simulink model "ADCS_GNC_Real_Simulation"  (R2025a)
settings: Solver=ode4  StartTime=0.0  StopTime=600  FixedStep=dt_sim  RelTol=1e-3
values from neighbouring files (symbols this model uses):
  Area_drag = 1.5    [ADCS_Real_Baseline.m]    (also in ADCS_Real_Baseline_Aerospace_Toolbox.m)
  Cd = 2.2    [ADCS_Real_Baseline.m]    (also in ADCS_Real_Baseline_Aerospace_Toolbox.m)
  cp_cg_offset_drag = [0.05; 0.02; -0.03]    [ADCS_Real_Baseline.m]    (also in ADCS_Real_Baseline_Aerospace_Toolbox.m)
  g0 = 9.80665    [ADCS_Real_Baseline.m]    (also in ADCS_Real_Baseline_Aerospace_Toolbox.m)
  gyro_bias_true = [1e-4; -2e-4; 1.5e-4]    [ADCS_Real_Baseline.m]    (also in ADCS_Real_Baseline_Aerospace_Toolbox.m)
  gyro_noise_sigma = 1e-5    (= 1e-05)    [ADCS_Real_Baseline.m]    (also in ADCS_Real_Baseline_Aerospace_Toolbox.m)
  I_inv = inv(I_tensor)    [ADCS_Real_Baseline.m]    (also in ADCS_Real_Baseline_Aerospace_Toolbox.m)
  I_tensor = diag([I_xx, I_yy, I_zz])    [ADCS_Real_Baseline.m]    (also in ADCS_Real_Baseline_Aerospace_Toolbox.m)
  Kd = diag(diag(2 * zeta * I_tensor * omega_n))    [ADCS_Real_Baseline.m]    (also in ADCS_Real_Baseline_Aerospace_Toolbox.m)
  Kp = diag(diag(I_tensor * omega_n^2))    [ADCS_Real_Baseline.m]    (also in ADCS_Real_Baseline_Aerospace_Toolbox.m)
  mtq_max_dipole = 15.0    (= 15)    [ADCS_Real_Baseline.m]    (also in ADCS_Real_Baseline_Aerospace_Toolbox.m)
  mtq_power_W_per_Am2 = 0.5    [ADCS_Real_Baseline.m]    (also in ADCS_Real_Baseline_Aerospace_Toolbox.m)
  mu_E = 398600.4418    [ADCS_Real_Baseline.m]    (also in ADCS_Real_Baseline_Aerospace_Toolbox.m)
  omega_init = C_BL_init * omega_orb_LVLH    [ADCS_Real_Baseline.m]    (also in ADCS_Real_Baseline_Aerospace_Toolbox.m)
  omega_orb_mag = sqrt(mu_E / r_orbit^3)    [ADCS_Real_Baseline.m]    (also in ADCS_Real_Baseline_Aerospace_Toolbox.m)
  q_init = q_init / norm(q_init)    [ADCS_Real_Baseline.m]    (also in ADCS_Real_Baseline_Aerospace_Toolbox.m)
  q_LVLH_ECI_init = q_LVLH_ECI_init / norm(q_LVLH_ECI_init)    [ADCS_Real_Baseline.m]    (also in ADCS_Real_Baseline_Aerospace_Toolbox.m)
  r_orbit = R_E + h_orbit    (= 7171)    [ADCS_Real_Baseline.m]    (also in ADCS_Real_Baseline_Aerospace_Toolbox.m)
  rho_atm = 1e-13    [ADCS_Real_Baseline.m]    (also in ADCS_Real_Baseline_Aerospace_Toolbox.m)
  rw_max_torque = 0.05    [ADCS_Real_Baseline.m]    (also in ADCS_Real_Baseline_Aerospace_Toolbox.m)
  rw_power_W_per_Nm = 50.0    (= 50)    [ADCS_Real_Baseline.m]    (also in ADCS_Real_Baseline_Aerospace_Toolbox.m)
  st_noise_sigma = 5e-4    (= 0.0005)    [ADCS_Real_Baseline.m]    (also in ADCS_Real_Baseline_Aerospace_Toolbox.m)
  thruster_arm = 0.5    [ADCS_Real_Baseline.m]    (also in ADCS_Real_Baseline_Aerospace_Toolbox.m)
  thruster_Isp = 65.0    (= 65)    [ADCS_Real_Baseline.m]    (also in ADCS_Real_Baseline_Aerospace_Toolbox.m)
  thruster_max_torque = thruster_force * thruster_arm    (= 0.5)    [ADCS_Real_Baseline.m]    (also in ADCS_Real_Baseline_Aerospace_Toolbox.m)
  V_orb = sqrt(mu_E*1e9 / (r_orbit*1e3))    [ADCS_Real_Baseline.m]    (also in ADCS_Real_Baseline_Aerospace_Toolbox.m)
(part 1 of 2)
settings Model: Creator=Simone  LastModifiedBy=Simone

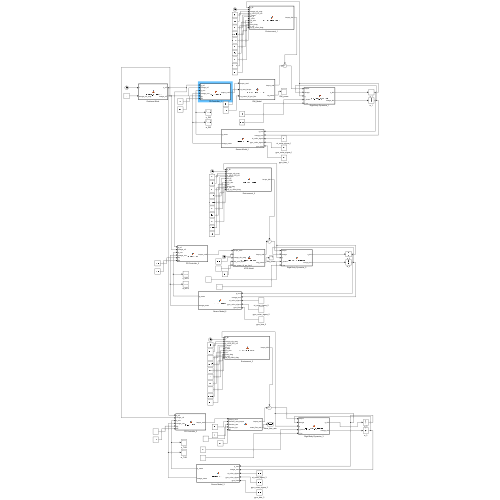
[thumbnail: Simulink's stored preview of the top-level diagram]
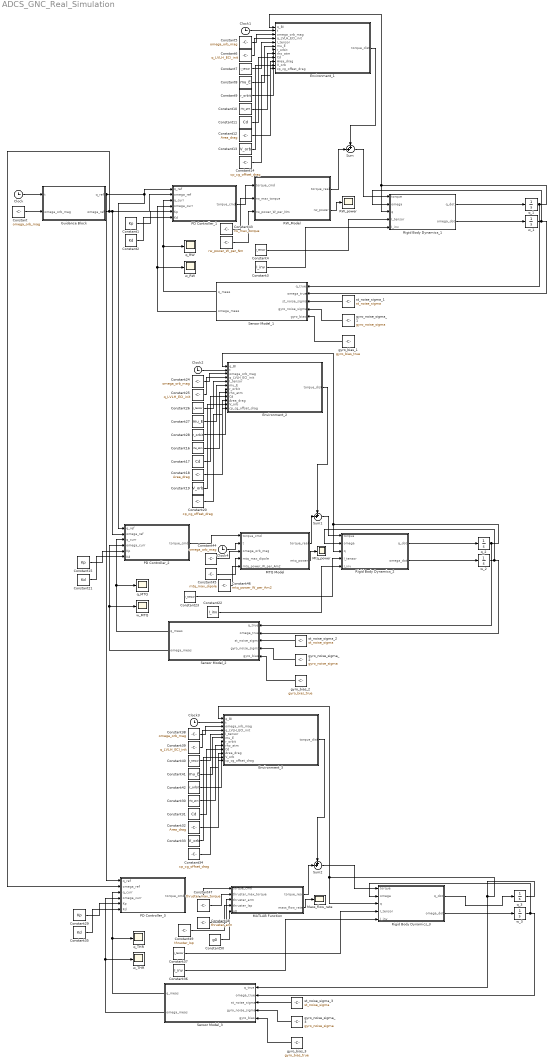
== system ADCS_GNC_Real_Simulation ==
  "                   " : Constant  Value=rw_power_W_per_Nm
  Clock{,1..4} (5 alike) : Clock
  Constant{,5,24,38,44} (5 alike) : Constant  Value=omega_orb_mag
  Constant1 : Constant  Value=Kp
  Constant10 : Constant  Value=rho_atm
  Constant11 : Constant  Value=Cd
  Constant12 : Constant  Value=Area_drag
  Constant13 : Constant  Value=V_orb
  Constant14 : Constant  Value=cp_cg_offset_drag
  Constant15 : Constant  Value=Kp
  Constant16 : Constant  Value=rho_atm
  Constant17 : Constant  Value=Cd
  Constant18 : Constant  Value=Area_drag
  Constant19 : Constant  Value=V_orb
  Constant2 : Constant  Value=Kd
  Constant20 : Constant  Value=cp_cg_offset_drag
  Constant21 : Constant  Value=Kd
  Constant22 : Constant  Value=I_inv
  Constant{4,7,23,26,37,40} (6 alike) : Constant  Value=I_tensor
  Constant25 : Constant  Value=q_LVLH_ECI_init
  Constant27 : Constant  Value=mu_E
  Constant28 : Constant  Value=r_orbit
  Constant29 : Constant  Value=Kp
  Constant3 : Constant  Value=I_inv
  Constant30 : Constant  Value=rho_atm
  Constant31 : Constant  Value=Cd
  Constant32 : Constant  Value=Area_drag
  Constant33 : Constant  Value=V_orb
  Constant34 : Constant  Value=cp_cg_offset_drag
  Constant35 : Constant  Value=Kd
  Constant36 : Constant  Value=I_inv
  Constant39 : Constant  Value=q_LVLH_ECI_init
  Constant41 : Constant  Value=mu_E
  Constant42 : Constant  Value=r_orbit
  Constant43 : Constant  Value=rw_max_torque
  Constant45 : Constant  Value=mtq_max_dipole
  Constant46 : Constant  Value=mtq_power_W_per_Am2
  Constant47 : Constant  Value=thruster_max_torque
  Constant48 : Constant  Value=thruster_arm
  Constant49 : Constant  Value=thruster_Isp
  Constant50 : Constant  Value=g0
  Constant6 : Constant  Value=q_LVLH_ECI_init
  Constant8 : Constant  Value=mu_E
  Constant9 : Constant  Value=r_orbit
  Environment_1 : MATLAB Function  TreatAsAtomicUnit=on
  Environment_2 : MATLAB Function  TreatAsAtomicUnit=on
  Environment_3 : MATLAB Function  TreatAsAtomicUnit=on
  Guidance Block : MATLAB Function  TreatAsAtomicUnit=on
  MATLAB Function : MATLAB Function  TreatAsAtomicUnit=on
  MTQ Model : MATLAB Function  TreatAsAtomicUnit=on
  Mass_flow_rate : Scope
      settings: ActiveDisplayYMinimum=-1  ActiveDisplayYMaximum=1  DataLoggingVariableName=out_mass_THR
  Mtq_power : Scope
      settings: ActiveDisplayYMinimum=-2.7921062281111855  ActiveDisplayYMaximum=25.310234025345686  DataLoggingVariableName=out_pwr_MTQ
  PD Controller_1 : MATLAB Function  TreatAsAtomicUnit=on
  PD Controller_2 : MATLAB Function  TreatAsAtomicUnit=on
  PD Controller_3 : MATLAB Function  TreatAsAtomicUnit=on
  RW_Model : MATLAB Function  TreatAsAtomicUnit=on
  RW_power : Scope
      settings: ActiveDisplayYMinimum=-0.049707954555951867  ActiveDisplayYMaximum=0.450202323670987  DataLoggingVariableName=out_pwr_RW
  Rigid Body Dynamics_1 : MATLAB Function  TreatAsAtomicUnit=on
  Rigid Body Dynamics_2 : MATLAB Function  TreatAsAtomicUnit=on
  Rigid Body Dynamics_3 : MATLAB Function  TreatAsAtomicUnit=on
  Sensor Model_1 : MATLAB Function  TreatAsAtomicUnit=on
  Sensor Model_2 : MATLAB Function  TreatAsAtomicUnit=on
  Sensor Model_3 : MATLAB Function  TreatAsAtomicUnit=on
  Sum : Sum  Inputs=++|
  Sum1 : Sum  Inputs=++|
  Sum2 : Sum  Inputs=++|
  gyro_bias_1 : Constant  Value=gyro_bias_true
  gyro_bias_2 : Constant  Value=gyro_bias_true
  gyro_bias_3 : Constant  Value=gyro_bias_true
  gyro_noise_sigma_1 : Constant  Value=gyro_noise_sigma
  gyro_noise_sigma_2 : Constant  Value=gyro_noise_sigma
  gyro_noise_sigma_3 : Constant  Value=gyro_noise_sigma
  q_1 : Integrator  InitialCondition=q_init
  q_2 : Integrator  InitialCondition=q_init
  q_3 : Integrator  InitialCondition=q_init
  q_MTQ : Scope
      settings: ActiveDisplayYMinimum=-0.90748752477080563  ActiveDisplayYMaximum=0.91859704888515026  DataLoggingVariableName=out_q_MTQ
  q_RW : Scope
      settings: ActiveDisplayYMinimum=-0.90748752477080563  ActiveDisplayYMaximum=0.91859704888515026  DataLoggingVariableName=out_q_RW
  q_THR : Scope
      settings: ActiveDisplayYMinimum=-0.90748752477080563  ActiveDisplayYMaximum=0.91859704888515026  DataLoggingVariableName=out_q_THR
  st_noise_sigma_1 : Constant  Value=st_noise_sigma
  st_noise_sigma_2 : Constant  Value=st_noise_sigma
  st_noise_sigma_3 : Constant  Value=st_noise_sigma
  w_1 : Integrator  InitialCondition=omega_init
  w_2 : Integrator  InitialCondition=omega_init
  w_3 : Integrator  InitialCondition=omega_init
  w_MTQ : Scope
      settings: ActiveDisplayYMinimum=-0.0048755943780988114  ActiveDisplayYMaximum=0.014930088485496639  DataLoggingVariableName=out_w_MTQ
  w_RW : Scope
      settings: ActiveDisplayYMinimum=-0.0048755943780988114  ActiveDisplayYMaximum=0.014930088485496639  DataLoggingVariableName=out_w_RW
  w_THR : Scope
      settings: ActiveDisplayYMinimum=-0.0048755943780988114  ActiveDisplayYMaximum=0.014930088485496639  DataLoggingVariableName=out_w_THR
  wires:
  Rigid Body Dynamics_1/1(q_dot) -> q_1/1
  Rigid Body Dynamics_1/2(omega_dot) -> w_1/1
  Clock/1 -> Guidance Block/1(t)
  Constant/1 -> Guidance Block/2(omega_orb_mag)
  Constant1/1 -> PD Controller_1/5(Kp)
  Constant2/1 -> PD Controller_1/6(Kd)
  Constant4/1 -> Rigid Body Dynamics_1/4(I_tensor)
  Constant3/1 -> Rigid Body Dynamics_1/5(I_inv)
  q_1/1 -> Rigid Body Dynamics_1/3(q), Environment_1/1(q_BI), Sensor Model_1/1(q_true)
  w_1/1 -> Rigid Body Dynamics_1/2(omega), Sensor Model_1/2(omega_true)
  st_noise_sigma_1/1 -> Sensor Model_1/3(st_noise_sigma)
  gyro_noise_sigma_1/1 -> Sensor Model_1/4(gyro_noise_sigma)
  gyro_bias_1/1 -> Sensor Model_1/5(gyro_bias)
  Sensor Model_1/1(q_meas) -> PD Controller_1/3(q_curr), q_RW/1
  Sensor Model_1/2(omega_meas) -> PD Controller_1/4(omega_curr), w_RW/1
  Clock1/1 -> Environment_1/2(t)
  Constant5/1 -> Environment_1/3(omega_orb_mag)
  Constant6/1 -> Environment_1/4(q_LVLH_ECI_init)
  Constant7/1 -> Environment_1/5(I_tensor)
  Constant8/1 -> Environment_1/6(mu_E)
  Constant9/1 -> Environment_1/7(r_orbit)
  Constant10/1 -> Environment_1/8(rho_atm)
  Constant11/1 -> Environment_1/9(Cd)
  Constant12/1 -> Environment_1/10(Area_drag)
  Constant13/1 -> Environment_1/11(V_orb)
  Constant14/1 -> Environment_1/12(cp_cg_offset_drag)
  Environment_1/1(torque_dist) -> Sum/1
  gyro_noise_sigma_2/1 -> Sensor Model_2/4(gyro_noise_sigma)
  st_noise_sigma_2/1 -> Sensor Model_2/3(st_noise_sigma)
  Sensor Model_2/1(q_meas) -> PD Controller_2/3(q_curr), q_MTQ/1
  Constant17/1 -> Environment_2/9(Cd)
  Constant20/1 -> Environment_2/12(cp_cg_offset_drag)
  Constant27/1 -> Environment_2/6(mu_E)
  Constant19/1 -> Environment_2/11(V_orb)
  Constant18/1 -> Environment_2/10(Area_drag)
  Constant26/1 -> Environment_2/5(I_tensor)
  Constant25/1 -> Environment_2/4(q_LVLH_ECI_init)
  gyro_bias_2/1 -> Sensor Model_2/5(gyro_bias)
  q_2/1 -> Rigid Body Dynamics_2/3(q), Environment_2/1(q_BI), Sensor Model_2/1(q_true)
  w_2/1 -> Rigid Body Dynamics_2/2(omega), Sensor Model_2/2(omega_true)
  Constant24/1 -> Environment_2/3(omega_orb_mag)
  Clock2/1 -> Environment_2/2(t)
  Constant23/1 -> Rigid Body Dynamics_2/4(I_tensor)
  Rigid Body Dynamics_2/1(q_dot) -> q_2/1
  Sensor Model_2/2(omega_meas) -> PD Controller_2/4(omega_curr), w_MTQ/1
  Constant16/1 -> Environment_2/8(rho_atm)
  Environment_2/1(torque_dist) -> Sum1/1
  Rigid Body Dynamics_2/2(omega_dot) -> w_2/1
  Constant15/1 -> PD Controller_2/5(Kp)
  Constant22/1 -> Rigid Body Dynamics_2/5(I_inv)
  Constant21/1 -> PD Controller_2/6(Kd)
  Constant28/1 -> Environment_2/7(r_orbit)
  gyro_noise_sigma_3/1 -> Sensor Model_3/4(gyro_noise_sigma)
  st_noise_sigma_3/1 -> Sensor Model_3/3(st_noise_sigma)
  Sensor Model_3/1(q_meas) -> PD Controller_3/3(q_curr), q_THR/1
  Constant31/1 -> Environment_3/9(Cd)
  Constant34/1 -> Environment_3/12(cp_cg_offset_drag)
  Constant41/1 -> Environment_3/6(mu_E)
  Constant33/1 -> Environment_3/11(V_orb)
  Constant32/1 -> Environment_3/10(Area_drag)
  Constant40/1 -> Environment_3/5(I_tensor)
  Constant39/1 -> Environment_3/4(q_LVLH_ECI_init)
  gyro_bias_3/1 -> Sensor Model_3/5(gyro_bias)
  q_3/1 -> Rigid Body Dynamics_3/3(q), Environment_3/1(q_BI), Sensor Model_3/1(q_true)
  w_3/1 -> Rigid Body Dynamics_3/2(omega), Sensor Model_3/2(omega_true)
  Constant38/1 -> Environment_3/3(omega_orb_mag)
  Clock3/1 -> Environment_3/2(t)
  Guidance Block/2(omega_ref) -> PD Controller_3/2(omega_ref), PD Controller_2/2(omega_ref), PD Controller_1/2(omega_ref)
  Constant37/1 -> Rigid Body Dynamics_3/4(I_tensor)
  Rigid Body Dynamics_3/1(q_dot) -> q_3/1
  Guidance Block/1(q_ref) -> PD Controller_3/1(q_ref), PD Controller_1/1(q_ref), PD Controller_2/1(q_ref)
  Sensor Model_3/2(omega_meas) -> PD Controller_3/4(omega_curr), w_THR/1
  Constant30/1 -> Environment_3/8(rho_atm)
  Environment_3/1(torque_dist) -> Sum2/1
  Rigid Body Dynamics_3/2(omega_dot) -> w_3/1
  Constant29/1 -> PD Controller_3/5(Kp)
  Constant36/1 -> Rigid Body Dynamics_3/5(I_inv)
  Constant35/1 -> PD Controller_3/6(Kd)
  Constant42/1 -> Environment_3/7(r_orbit)
  PD Controller_1/1(torque_cmd) -> RW_Model/1(torque_cmd)
  Constant43/1 -> RW_Model/2(rw_max_torque)
  "                   "/1 -> RW_Model/3(rw_power_W_per_Nm)
  RW_Model/1(torque_real) -> Sum/2
  Sum/1 -> Rigid Body Dynamics_1/1(torque)
  RW_Model/2(rw_power) -> RW_power/1
  Constant44/1 -> MTQ Model/3(omega_orb_mag)
  Constant45/1 -> MTQ Model/4(mtq_max_dipole)
  Constant46/1 -> MTQ Model/5(mtq_power_W_per_Am2)
  Clock4/1 -> MTQ Model/2(t)
  PD Controller_2/1(torque_cmd) -> MTQ Model/1(torque_cmd)
  MTQ Model/1(torque_real) -> Sum1/2
  Sum1/1 -> Rigid Body Dynamics_2/1(torque)
  MTQ Model/2(mtq_power) -> Mtq_power/1
  Constant47/1 -> MATLAB Function/2(thruster_max_torque)
  Constant48/1 -> MATLAB Function/3(thruster_arm)
  Constant49/1 -> MATLAB Function/4(thruster_Isp)
  Constant50/1 -> MATLAB Function/5(g0)
  PD Controller_3/1(torque_cmd) -> MATLAB Function/1(torque_cmd)
  MATLAB Function/1(torque_real) -> Sum2/2
  Sum2/1 -> Rigid Body Dynamics_3/1(torque)
  MATLAB Function/2(mass_flow_rate) -> Mass_flow_rate/1

== matlab function ADCS_GNC_Real_Simulation/Rigid Body Dynamics_2 ==
  data: torque input; q_dot output; omega input; q input; I_tensor input; I_inv input; omega_dot output
function [q_dot, omega_dot] = rigid_body_dynamics(torque, omega, q, I_tensor, I_inv)
% =========================================================================
% RIGID BODY ROTATIONAL DYNAMICS + QUATERNION KINEMATICS
% =========================================================================
% Purpose:
%   Simulate the rotational motion of the spacecraft.
%
% Inputs:
%   torque   : Applied body torque [Tx; Ty; Tz] [Nm]
%              expressed in BODY coordinates
%
%   omega    : Body angular velocity [p; q; r] [rad/s]
%              expressed in BODY coordinates
%
%   q        : Attitude quaternion [qw; qx; qy; qz]
%              BODY attitude with respect to ECI
%
%   I_tensor : Spacecraft inertia tensor [kg*m^2]
%
%   I_inv    : Inverse inertia tensor [1/(kg*m^2)]
%
% Outputs:
%   q_dot    : Quaternion derivative
%
%   omega_dot: Body angular acceleration [rad/s^2]
%
% =========================================================================
% Dynamic equation:
%
%   I * omega_dot + omega x (I*omega) = torque
%
% Therefore:
%
%   omega_dot = I^-1 * [torque - omega x (I*omega)]
%
% =========================================================================


% -------------------------------------------------------------------------
% 1. INITIALIZE OUTPUTS
% -------------------------------------------------------------------------

q_dot     = zeros(4,1);
omega_dot = zeros(3,1);


% -------------------------------------------------------------------------
% 2. NORMALIZE QUATERNION FOR KINEMATIC CALCULATION
% -------------------------------------------------------------------------
% Numerical integration can cause a small drift in quaternion norm.
%
% We normalize the quaternion before calculating q_dot.
% This does not change the physical attitude.

q_norm = norm(q);

if q_norm > 1e-12
    q_unit = q / q_norm;
else
    % Safety fallback
    q_unit = [1; 0; 0; 0];
end


% -------------------------------------------------------------------------
% 3. ANGULAR MOMENTUM
% -------------------------------------------------------------------------
% Angular momentum:
%
%   H = I * omega

H = I_tensor * omega;


% -------------------------------------------------------------------------
% 4. GYROSCOPIC CROSS PRODUCT
% -------------------------------------------------------------------------
% Calculate:
%
%   omega x H
%
% where:
%
%   H = I * omega

cross_omega_H = [ ...
    omega(2)*H(3) - omega(3)*H(2);
    omega(3)*H(1) - omega(1)*H(3);
    omega(1)*H(2) - omega(2)*H(1) ];


% -------------------------------------------------------------------------
% 5. EULER ROTATIONAL DYNAMICS
% -------------------------------------------------------------------------
% Equation:
%
%   I * omega_dot = torque - omega x (I*omega)
%
% Therefore:
%
%   omega_dot = I^-1 * [torque - omega x (I*omega)]

omega_dot = I_inv * ( ...
    torque - cross_omega_H );


% -------------------------------------------------------------------------
% 6. BODY ANGULAR RATES
% -------------------------------------------------------------------------
% The three components are:
%
%   omega = [p; q; r]

p = omega(1);
q_rate = omega(2);
r = omega(3);


% -------------------------------------------------------------------------
% 7. QUATERNION KINEMATICS
% -------------------------------------------------------------------------
% Quaternion convention:
%
%   q = [qw; qx; qy; qz]
%
% with body angular velocity:
%
%   omega = [p; q; r]
%
% Quaternion differential equation:
%
%   q_dot = 0.5 * Omega(omega) * q
%
% where:
%
%       [ 0  -p  -q  -r ]
%       [ p   0   r  -q ]
% Omega=[ q  -r   0   p ]
%       [ r   q  -p   0 ]

Omega_mat = [ ...
     0,     -p,      -q_rate, -r;
     p,      0,       r,      -q_rate;
     q_rate,-r,       0,       p;
     r,      q_rate, -p,       0 ];


% Quaternion derivative
q_dot = 0.5 * Omega_mat * q_unit;


% -------------------------------------------------------------------------
% 8. END
% -------------------------------------------------------------------------

end

== matlab function ADCS_GNC_Real_Simulation/Sensor Model_2 ==
  settings: updateMethod=DISCRETE
  data: q_true input; q_meas output; omega_true input; st_noise_sigma input; gyro_noise_sigma input; gyro_bias input; omega_meas output
function [q_meas, omega_meas] = sensor_model(q_true, omega_true, st_noise_sigma, gyro_noise_sigma, gyro_bias)
    % =====================================================================
    % SENSOR MODEL (STAR TRACKER & GYROSCOPES)
    % Inputs:
    %   q_true           : 4x1 True attitude quaternion from dynamics
    %   omega_true       : 3x1 True angular velocity from dynamics [rad/s]
    %   st_noise_sigma   : Scalar, Star Tracker noise standard deviation [rad]
    %   gyro_noise_sigma : Scalar, Gyroscope noise standard deviation [rad/s]
    %   gyro_bias        : 3x1 Gyroscope constant thermal drift [rad/s]
    %
    % Outputs:
    %   q_meas           : 4x1 Measured (noisy) quaternion
    %   omega_meas       : 3x1 Measured (noisy) angular velocity
    % =====================================================================

    % 1. GYROSCOPE MODEL (Angular Velocity)
    % Equation: w_meas = w_true + bias + noise
    % We use randn(3,1) to generate normally distributed Gaussian white noise.
    gyro_noise = gyro_noise_sigma * randn(3, 1);
    omega_meas = omega_true + gyro_bias + gyro_noise;

    % 2. STAR TRACKER MODEL (Attitude Quaternion)
    % Instead of adding noise directly to quaternion components (which breaks 
    % its properties), we generate a small random error rotation vector.
    
    % Small angle error on 3 axes [rad]
    err_angles = st_noise_sigma * randn(3, 1);
    
    % Convert small angle error to an error quaternion (Small Angle Approximation)
    % q_err = [1; theta_x/2; theta_y/2; theta_z/2]
    q_err = [1; 0.5 * err_angles(1); 0.5 * err_angles(2); 0.5 * err_angles(3)];
    q_err = q_err / norm(q_err); % Normalize just to be safe
    
    % Apply the error rotation to the true quaternion (Hamilton product)
    % q_meas = q_true * q_err
    qw = q_true(1); qx = q_true(2); qy = q_true(3); qz = q_true(4);
    ew = q_err(1);  ex = q_err(2);  ey = q_err(3);  ez = q_err(4);
    
    q_meas = [ ...
        qw*ew - qx*ex - qy*ey - qz*ez;
        qw*ex + qx*ew + qy*ez - qz*ey;
        qw*ey - qx*ez + qy*ew + qz*ex;
        qw*ez + qx*ey - qy*ex + qz*ew ];
        
    % Final normalization to ensure the controller receives a valid unit quaternion
    q_meas = q_meas / norm(q_meas);
end

== matlab function ADCS_GNC_Real_Simulation/Environment_3 ==
  data: q_BI input; torque_dist output; t input; omega_orb_mag input; q_LVLH_ECI_init input; I_tensor input; mu_E input; r_orbit input; rho_atm input; Cd input; Area_drag input; V_orb input; cp_cg_offset_drag input
function torque_dist = environment_model(q_BI, t, omega_orb_mag, q_LVLH_ECI_init, I_tensor, mu_E, r_orbit, rho_atm, Cd, Area_drag, V_orb, cp_cg_offset_drag)
    % =====================================================================
    % ENVIRONMENTAL DISTURBANCES MODEL
    % Calculates Gravity Gradient and Aerodynamic Drag torques in BODY frame.
    % =====================================================================
    
    % 1. Calculate current LVLH to ECI quaternion (Orbit evolution)
    theta_orb = -omega_orb_mag * t;
    q_orb_rot = [cos(theta_orb/2); 0; sin(theta_orb/2); 0];
    
    % Hamilton product: q_LI_curr = q_orb_rot * q_LVLH_ECI_init
    qw1 = q_orb_rot(1); qx1 = q_orb_rot(2); qy1 = q_orb_rot(3); qz1 = q_orb_rot(4);
    qw2 = q_LVLH_ECI_init(1); qx2 = q_LVLH_ECI_init(2); qy2 = q_LVLH_ECI_init(3); qz2 = q_LVLH_ECI_init(4);
    q_LI_curr = [ ...
        qw1*qw2 - qx1*qx2 - qy1*qy2 - qz1*qz2;
        qw1*qx2 + qx1*qw2 + qy1*qz2 - qz1*qy2;
        qw1*qy2 - qx1*qz2 + qy1*qw2 + qz1*qx2;
        qw1*qz2 + qx1*qy2 - qy1*qx2 + qz1*qw2 ];
        
    % 2. Calculate BODY to LVLH quaternion: q_BL = q_BI * q_LI_curr^(-1)
    q_LI_conj = [q_LI_curr(1); -q_LI_curr(2); -q_LI_curr(3); -q_LI_curr(4)];
    
    qw1 = q_BI(1); qx1 = q_BI(2); qy1 = q_BI(3); qz1 = q_BI(4);
    qw2 = q_LI_conj(1); qx2 = q_LI_conj(2); qy2 = q_LI_conj(3); qz2 = q_LI_conj(4);
    q_BL = [ ...
        qw1*qw2 - qx1*qx2 - qy1*qy2 - qz1*qz2;
        qw1*qx2 + qx1*qw2 + qy1*qz2 - qz1*qy2;
        qw1*qy2 - qx1*qz2 + qy1*qw2 + qz1*qx2;
        qw1*qz2 + qx1*qy2 - qy1*qx2 + qz1*qw2 ];
    q_BL = q_BL / norm(q_BL);
    
    % 3. DCM from LVLH to BODY
    qw = q_BL(1); qx = q_BL(2); qy = q_BL(3); qz = q_BL(4);
    C_BL = [ ...
        1 - 2*(qy^2 + qz^2),     2*(qx*qy + qw*qz),       2*(qx*qz - qw*qy);
        2*(qx*qy - qw*qz),       1 - 2*(qx^2 + qz^2),     2*(qy*qz + qw*qx);
        2*(qx*qz + qw*qy),       2*(qy*qz - qw*qx),       1 - 2*(qx^2 + qy^2) ];
        
    % ---------------------------------------------------------------------
    % A) GRAVITY GRADIENT TORQUE
    % Nadir vector in LVLH is X-axis [1; 0; 0]
    % ---------------------------------------------------------------------
    u_nadir_LVLH = [1; 0; 0];
    u_nadir_BODY = C_BL * u_nadir_LVLH;
    
    % tau_gg = 3 * (mu/r^3) * (u_nadir x I * u_nadir)
    mu_m3 = mu_E * 1e9;         % Convert km^3/s^2 to m^3/s^2
    r_m = r_orbit * 1e3;        % Convert km to m
    tau_gg = 3 * (mu_m3) / (r_m^3) * cross(u_nadir_BODY, I_tensor * u_nadir_BODY);
    
    % ---------------------------------------------------------------------
    % B) AERODYNAMIC DRAG TORQUE
    % Satellite moves along LVLH +Y. So the incoming wind is -Y [0; -1; 0]
    % ---------------------------------------------------------------------
    u_wind_LVLH = [0; -1; 0];
    u_wind_BODY = C_BL * u_wind_LVLH;
    
    % F_drag = 0.5 * rho * Cd * A * V^2 * u_wind
    F_drag_mag = 0.5 * rho_atm * Cd * Area_drag * V_orb^2;
    F_drag_BODY = F_drag_mag * u_wind_BODY;
    
    % tau_drag = offset x F_drag
    tau_drag = cross(cp_cg_offset_drag, F_drag_BODY);
    
    % ---------------------------------------------------------------------
    % TOTAL DISTURBANCE TORQUE
    % ---------------------------------------------------------------------
    torque_dist = tau_gg + tau_drag;
end

== matlab function ADCS_GNC_Real_Simulation/PD Controller_3 ==
  data: q_ref input; torque_cmd output; omega_ref input; q_curr input; omega_curr input; Kp input; Kd input
function torque_cmd = pd_controller(q_ref, omega_ref, q_curr, omega_curr, Kp, Kd)
% =========================================================================
% QUATERNION PD ATTITUDE CONTROLLER
% =========================================================================
% Purpose:
%   Compute the spacecraft control torque required to track the desired
%   attitude and angular velocity.
%
% Inputs:
%   q_ref      : Desired quaternion [qw; qx; qy; qz]
%                BODY attitude with respect to ECI
%
%   omega_ref  : Desired angular velocity [p; q; r]
%                expressed in BODY coordinates
%
%   q_curr     : Current quaternion [qw; qx; qy; qz]
%                BODY attitude with respect to ECI
%
%   omega_curr : Current body angular velocity [p; q; r]
%                expressed in BODY coordinates
%
%   Kp         : Proportional gain matrix
%   Kd         : Derivative gain matrix
%
% Output:
%   torque_cmd : Control torque [Tx; Ty; Tz] in BODY coordinates [Nm]
%
% Quaternion convention:
%   Scalar first: [qw; qx; qy; qz]
%
% =========================================================================


% -------------------------------------------------------------------------
% 1. INITIALIZE OUTPUT
% -------------------------------------------------------------------------

torque_cmd = zeros(3,1);


% -------------------------------------------------------------------------
% 2. NORMALIZE QUATERNIONS
% -------------------------------------------------------------------------
% A valid attitude quaternion must have unit norm.
%
% Normalization also prevents numerical integration errors from
% affecting the attitude error calculation.

q_curr_norm = norm(q_curr);
q_ref_norm  = norm(q_ref);

if q_curr_norm > 1e-12
    q_curr = q_curr / q_curr_norm;
end

if q_ref_norm > 1e-12
    q_ref = q_ref / q_ref_norm;
end


% -------------------------------------------------------------------------
% 3. CURRENT QUATERNION CONJUGATE
% -------------------------------------------------------------------------
% For a unit quaternion:
%
%   q_inverse = conjugate(q)
%
% Therefore:
%
%   q_curr_conj = [qw; -qx; -qy; -qz]

q_curr_conj = [ ...
     q_curr(1);
    -q_curr(2);
    -q_curr(3);
    -q_curr(4) ];


% -------------------------------------------------------------------------
% 4. ATTITUDE ERROR QUATERNION
% -------------------------------------------------------------------------
% We calculate:
%
%   q_err = conjugate(q_curr) * q_ref
%
% With the present convention, the vector part of q_err represents
% the rotation required to move the CURRENT attitude toward the
% REFERENCE attitude, expressed in the current/body coordinates.
%
% This is convenient because the control torque is also expressed
% in BODY coordinates.

% Current quaternion
qc_w = q_curr_conj(1);
qc_x = q_curr_conj(2);
qc_y = q_curr_conj(3);
qc_z = q_curr_conj(4);

% Reference quaternion
qr_w = q_ref(1);
qr_x = q_ref(2);
qr_y = q_ref(3);
qr_z = q_ref(4);


% Hamilton product:
% q_err = q_curr_conj * q_ref

q_err_w = ...
    qc_w*qr_w ...
    - qc_x*qr_x ...
    - qc_y*qr_y ...
    - qc_z*qr_z;

q_err_x = ...
    qc_w*qr_x ...
    + qc_x*qr_w ...
    + qc_y*qr_z ...
    - qc_z*qr_y;

q_err_y = ...
    qc_w*qr_y ...
    - qc_x*qr_z ...
    + qc_y*qr_w ...
    + qc_z*qr_x;

q_err_z = ...
    qc_w*qr_z ...
    + qc_x*qr_y ...
    - qc_y*qr_x ...
    + qc_z*qr_w;


% Vector part of the attitude error
q_err_vec = [ ...
    q_err_x;
    q_err_y;
    q_err_z ];


% -------------------------------------------------------------------------
% 5. SHORTEST-ROTATION PATH
% -------------------------------------------------------------------------
% q and -q represent the same physical attitude.
%
% If the scalar part of the error quaternion is negative, flip the
% vector part so that the controller follows the shortest rotation.

if q_err_w < 0
    q_err_vec = -q_err_vec;
end


% -------------------------------------------------------------------------
% 6. ANGULAR VELOCITY ERROR
% -------------------------------------------------------------------------
% Both omega_curr and omega_ref are expressed in BODY coordinates.
%
% Therefore they can be directly subtracted.

delta_omega = omega_curr - omega_ref;


% -------------------------------------------------------------------------
% 7. QUATERNION PD CONTROL LAW
% -------------------------------------------------------------------------
% Control law:
%
%   torque = Kp * q_error_vector
%            - Kd * angular_velocity_error
%
% The positive proportional sign is consistent with the definition:
%
%   q_err = conjugate(q_curr) * q_ref
%
% A positive q_err vector indicates the direction toward the target.

torque_cmd = Kp * q_err_vec ...
           - Kd * delta_omega;


% -------------------------------------------------------------------------
% 8. OUTPUT
% -------------------------------------------------------------------------
% torque_cmd is expressed in BODY coordinates:
%
%   [Tx; Ty; Tz] [Nm]

end

== matlab function ADCS_GNC_Real_Simulation/Rigid Body Dynamics_3 ==
  data: torque input; q_dot output; omega input; q input; I_tensor input; I_inv input; omega_dot output
function [q_dot, omega_dot] = rigid_body_dynamics(torque, omega, q, I_tensor, I_inv)
% =========================================================================
% RIGID BODY ROTATIONAL DYNAMICS + QUATERNION KINEMATICS
% =========================================================================
% Purpose:
%   Simulate the rotational motion of the spacecraft.
%
% Inputs:
%   torque   : Applied body torque [Tx; Ty; Tz] [Nm]
%              expressed in BODY coordinates
%
%   omega    : Body angular velocity [p; q; r] [rad/s]
%              expressed in BODY coordinates
%
%   q        : Attitude quaternion [qw; qx; qy; qz]
%              BODY attitude with respect to ECI
%
%   I_tensor : Spacecraft inertia tensor [kg*m^2]
%
%   I_inv    : Inverse inertia tensor [1/(kg*m^2)]
%
% Outputs:
%   q_dot    : Quaternion derivative
%
%   omega_dot: Body angular acceleration [rad/s^2]
%
% =========================================================================
% Dynamic equation:
%
%   I * omega_dot + omega x (I*omega) = torque
%
% Therefore:
%
%   omega_dot = I^-1 * [torque - omega x (I*omega)]
%
% =========================================================================


% -------------------------------------------------------------------------
% 1. INITIALIZE OUTPUTS
% -------------------------------------------------------------------------

q_dot     = zeros(4,1);
omega_dot = zeros(3,1);


% -------------------------------------------------------------------------
% 2. NORMALIZE QUATERNION FOR KINEMATIC CALCULATION
% -------------------------------------------------------------------------
% Numerical integration can cause a small drift in quaternion norm.
%
% We normalize the quaternion before calculating q_dot.
% This does not change the physical attitude.

q_norm = norm(q);

if q_norm > 1e-12
    q_unit = q / q_norm;
else
    % Safety fallback
    q_unit = [1; 0; 0; 0];
end


% -------------------------------------------------------------------------
% 3. ANGULAR MOMENTUM
% -------------------------------------------------------------------------
% Angular momentum:
%
%   H = I * omega

H = I_tensor * omega;


% -------------------------------------------------------------------------
% 4. GYROSCOPIC CROSS PRODUCT
% -------------------------------------------------------------------------
% Calculate:
%
%   omega x H
%
% where:
%
%   H = I * omega

cross_omega_H = [ ...
    omega(2)*H(3) - omega(3)*H(2);
    omega(3)*H(1) - omega(1)*H(3);
    omega(1)*H(2) - omega(2)*H(1) ];


% -------------------------------------------------------------------------
% 5. EULER ROTATIONAL DYNAMICS
% -------------------------------------------------------------------------
% Equation:
%
%   I * omega_dot = torque - omega x (I*omega)
%
% Therefore:
%
%   omega_dot = I^-1 * [torque - omega x (I*omega)]

omega_dot = I_inv * ( ...
    torque - cross_omega_H );


% -------------------------------------------------------------------------
% 6. BODY ANGULAR RATES
% -------------------------------------------------------------------------
% The three components are:
%
%   omega = [p; q; r]

p = omega(1);
q_rate = omega(2);
r = omega(3);


% -------------------------------------------------------------------------
% 7. QUATERNION KINEMATICS
% -------------------------------------------------------------------------
% Quaternion convention:
%
%   q = [qw; qx; qy; qz]
%
% with body angular velocity:
%
%   omega = [p; q; r]
%
% Quaternion differential equation:
%
%   q_dot = 0.5 * Omega(omega) * q
%
% where:
%
%       [ 0  -p  -q  -r ]
%       [ p   0   r  -q ]
% Omega=[ q  -r   0   p ]
%       [ r   q  -p   0 ]

Omega_mat = [ ...
     0,     -p,      -q_rate, -r;
     p,      0,       r,      -q_rate;
     q_rate,-r,       0,       p;
     r,      q_rate, -p,       0 ];


% Quaternion derivative
q_dot = 0.5 * Omega_mat * q_unit;


% -------------------------------------------------------------------------
% 8. END
% -------------------------------------------------------------------------

end

== matlab function ADCS_GNC_Real_Simulation/Sensor Model_3 ==
  settings: updateMethod=DISCRETE
  data: q_true input; q_meas output; omega_true input; st_noise_sigma input; gyro_noise_sigma input; gyro_bias input; omega_meas output
function [q_meas, omega_meas] = sensor_model(q_true, omega_true, st_noise_sigma, gyro_noise_sigma, gyro_bias)
    % =====================================================================
    % SENSOR MODEL (STAR TRACKER & GYROSCOPES)
    % Inputs:
    %   q_true           : 4x1 True attitude quaternion from dynamics
    %   omega_true       : 3x1 True angular velocity from dynamics [rad/s]
    %   st_noise_sigma   : Scalar, Star Tracker noise standard deviation [rad]
    %   gyro_noise_sigma : Scalar, Gyroscope noise standard deviation [rad/s]
    %   gyro_bias        : 3x1 Gyroscope constant thermal drift [rad/s]
    %
    % Outputs:
    %   q_meas           : 4x1 Measured (noisy) quaternion
    %   omega_meas       : 3x1 Measured (noisy) angular velocity
    % =====================================================================

    % 1. GYROSCOPE MODEL (Angular Velocity)
    % Equation: w_meas = w_true + bias + noise
    % We use randn(3,1) to generate normally distributed Gaussian white noise.
    gyro_noise = gyro_noise_sigma * randn(3, 1);
    omega_meas = omega_true + gyro_bias + gyro_noise;

    % 2. STAR TRACKER MODEL (Attitude Quaternion)
    % Instead of adding noise directly to quaternion components (which breaks 
    % its properties), we generate a small random error rotation vector.
    
    % Small angle error on 3 axes [rad]
    err_angles = st_noise_sigma * randn(3, 1);
    
    % Convert small angle error to an error quaternion (Small Angle Approximation)
    % q_err = [1; theta_x/2; theta_y/2; theta_z/2]
    q_err = [1; 0.5 * err_angles(1); 0.5 * err_angles(2); 0.5 * err_angles(3)];
    q_err = q_err / norm(q_err); % Normalize just to be safe
    
    % Apply the error rotation to the true quaternion (Hamilton product)
    % q_meas = q_true * q_err
    qw = q_true(1); qx = q_true(2); qy = q_true(3); qz = q_true(4);
    ew = q_err(1);  ex = q_err(2);  ey = q_err(3);  ez = q_err(4);
    
    q_meas = [ ...
        qw*ew - qx*ex - qy*ey - qz*ez;
        qw*ex + qx*ew + qy*ez - qz*ey;
        qw*ey - qx*ez + qy*ew + qz*ex;
        qw*ez + qx*ey - qy*ex + qz*ew ];
        
    % Final normalization to ensure the controller receives a valid unit quaternion
    q_meas = q_meas / norm(q_meas);
end

== matlab function ADCS_GNC_Real_Simulation/PD Controller_1 ==
  data: q_ref input; torque_cmd output; omega_ref input; q_curr input; omega_curr input; Kp input; Kd input
function torque_cmd = pd_controller(q_ref, omega_ref, q_curr, omega_curr, Kp, Kd)
% =========================================================================
% QUATERNION PD ATTITUDE CONTROLLER
% =========================================================================
% Purpose:
%   Compute the spacecraft control torque required to track the desired
%   attitude and angular velocity.
%
% Inputs:
%   q_ref      : Desired quaternion [qw; qx; qy; qz]
%                BODY attitude with respect to ECI
%
%   omega_ref  : Desired angular velocity [p; q; r]
%                expressed in BODY coordinates
%
%   q_curr     : Current quaternion [qw; qx; qy; qz]
%                BODY attitude with respect to ECI
%
%   omega_curr : Current body angular velocity [p; q; r]
%                expressed in BODY coordinates
%
%   Kp         : Proportional gain matrix
%   Kd         : Derivative gain matrix
%
% Output:
%   torque_cmd : Control torque [Tx; Ty; Tz] in BODY coordinates [Nm]
%
% Quaternion convention:
%   Scalar first: [qw; qx; qy; qz]
%
% =========================================================================


% -------------------------------------------------------------------------
% 1. INITIALIZE OUTPUT
% -------------------------------------------------------------------------

torque_cmd = zeros(3,1);


% -------------------------------------------------------------------------
% 2. NORMALIZE QUATERNIONS
% -------------------------------------------------------------------------
% A valid attitude quaternion must have unit norm.
%
% Normalization also prevents numerical integration errors from
% affecting the attitude error calculation.

q_curr_norm = norm(q_curr);
q_ref_norm  = norm(q_ref);

if q_curr_norm > 1e-12
    q_curr = q_curr / q_curr_norm;
end

if q_ref_norm > 1e-12
    q_ref = q_ref / q_ref_norm;
end


% -------------------------------------------------------------------------
% 3. CURRENT QUATERNION CONJUGATE
% -------------------------------------------------------------------------
% For a unit quaternion:
%
%   q_inverse = conjugate(q)
%
% Therefore:
%
%   q_curr_conj = [qw; -qx; -qy; -qz]

q_curr_conj = [ ...
     q_curr(1);
    -q_curr(2);
    -q_curr(3);
    -q_curr(4) ];


% -------------------------------------------------------------------------
% 4. ATTITUDE ERROR QUATERNION
% -------------------------------------------------------------------------
% We calculate:
%
%   q_err = conjugate(q_curr) * q_ref
%
% With the present convention, the vector part of q_err represents
% the rotation required to move the CURRENT attitude toward the
% REFERENCE attitude, expressed in the current/body coordinates.
%
% This is convenient because the control torque is also expressed
% in BODY coordinates.

% Current quaternion
qc_w = q_curr_conj(1);
qc_x = q_curr_conj(2);
qc_y = q_curr_conj(3);
qc_z = q_curr_conj(4);

% Reference quaternion
qr_w = q_ref(1);
qr_x = q_ref(2);
qr_y = q_ref(3);
qr_z = q_ref(4);


% Hamilton product:
% q_err = q_curr_conj * q_ref

q_err_w = ...
    qc_w*qr_w ...
    - qc_x*qr_x ...
    - qc_y*qr_y ...
    - qc_z*qr_z;

q_err_x = ...
    qc_w*qr_x ...
    + qc_x*qr_w ...
    + qc_y*qr_z ...
    - qc_z*qr_y;

q_err_y = ...
    qc_w*qr_y ...
    - qc_x*qr_z ...
    + qc_y*qr_w ...
    + qc_z*qr_x;

q_err_z = ...
    qc_w*qr_z ...
    + qc_x*qr_y ...
    - qc_y*qr_x ...
    + qc_z*qr_w;


% Vector part of the attitude error
q_err_vec = [ ...
    q_err_x;
    q_err_y;
    q_err_z ];


% -------------------------------------------------------------------------
% 5. SHORTEST-ROTATION PATH
% -------------------------------------------------------------------------
% q and -q represent the same physical attitude.
%
% If the scalar part of the error quaternion is negative, flip the
% vector part so that the controller follows the shortest rotation.

if q_err_w < 0
    q_err_vec = -q_err_vec;
end


% -------------------------------------------------------------------------
% 6. ANGULAR VELOCITY ERROR
% -------------------------------------------------------------------------
% Both omega_curr and omega_ref are expressed in BODY coordinates.
%
% Therefore they can be directly subtracted.

delta_omega = omega_curr - omega_ref;


% -------------------------------------------------------------------------
% 7. QUATERNION PD CONTROL LAW
% -------------------------------------------------------------------------
% Control law:
%
%   torque = Kp * q_error_vector
%            - Kd * angular_velocity_error
%
% The positive proportional sign is consistent with the definition:
%
%   q_err = conjugate(q_curr) * q_ref
%
% A positive q_err vector indicates the direction toward the target.

torque_cmd = Kp * q_err_vec ...
           - Kd * delta_omega;


% -------------------------------------------------------------------------
% 8. OUTPUT
% -------------------------------------------------------------------------
% torque_cmd is expressed in BODY coordinates:
%
%   [Tx; Ty; Tz] [Nm]

end

== matlab function ADCS_GNC_Real_Simulation/RW_Model ==
  data: torque_cmd input; torque_real output; rw_max_torque input; rw_power_W_per_Nm input; rw_power output
function [torque_real, rw_power] = reaction_wheels_model(torque_cmd, rw_max_torque, rw_power_W_per_Nm)
    % =====================================================================
    % REACTION WHEELS ACTUATOR MODEL
    % Simulates physical torque saturation and power consumption.
    % =====================================================================
    
    torque_real = zeros(3,1);
    
    % 1. TORQUE SATURATION (Hardware limits)
    % The wheels cannot provide more than 'rw_max_torque' per axis.
    for i = 1:3
        if torque_cmd(i) > rw_max_torque
            torque_real(i) = rw_max_torque;
        elseif torque_cmd(i) < -rw_max_torque
            torque_real(i) = -rw_max_torque;
        else
            torque_real(i) = torque_cmd(i);
        end
    end
    
    % 2. POWER CONSUMPTION BUDGET [Watts]
    % Simplified model: Power is linearly proportional to the torque provided.
    rw_power = sum(abs(torque_real)) * rw_power_W_per_Nm;
    
end

== matlab function ADCS_GNC_Real_Simulation/MTQ Model ==
  data: torque_cmd input; torque_real output; t input; omega_orb_mag input; mtq_max_dipole input; mtq_power_W_per_Am2 input; mtq_power output
function [torque_real, mtq_power] = magnetorquer_model(torque_cmd, t, omega_orb_mag, mtq_max_dipole, mtq_power_W_per_Am2)
    % =====================================================================
    % MAGNETORQUER ACTUATOR MODEL
    % Implements the Cross-Product Control Law and physical limitations.
    % =====================================================================
    
    % 1. MOCK EARTH MAGNETIC FIELD (B) IN BODY FRAME [Tesla]
    % For this trade-off, we simulate a realistic B-field that oscillates 
    % as the satellite travels along its orbit.
    B_mag = 40e-6; % ~40 microTesla in LEO
    B_body = B_mag * [sin(omega_orb_mag * t); cos(omega_orb_mag * t); 0.5];
    
    % 2. IDEAL DIPOLE COMMAND (Cross-Product Law)
    % Formula: m = (B x tau_cmd) / |B|^2
    % This calculates the required dipole to approximate the requested torque.
    m_cmd = cross(B_body, torque_cmd) / (norm(B_body)^2 + 1e-12);
    
    % 3. SATURATION (Hardware limits)
    m_real = zeros(3,1);
    for i = 1:3
        if m_cmd(i) > mtq_max_dipole
            m_real(i) = mtq_max_dipole;
        elseif m_cmd(i) < -mtq_max_dipole
            m_real(i) = -mtq_max_dipole;
        else
            m_real(i) = m_cmd(i);
        end
    end
    
    % 4. REAL TORQUE GENERATED
    % The actual torque applied to the spacecraft: tau = m x B
    torque_real = cross(m_real, B_body);
    
    % 5. POWER CONSUMPTION BUDGET [Watts]
    mtq_power = sum(abs(m_real)) * mtq_power_W_per_Am2;
end

== matlab function ADCS_GNC_Real_Simulation/MATLAB Function ==
  data: torque_cmd input; torque_real output; thruster_max_torque input; thruster_arm input; thruster_Isp input; g0 input; mass_flow_rate output
function [torque_real, mass_flow_rate] = thrusters_model(torque_cmd, thruster_max_torque, thruster_arm, thruster_Isp, g0)
    % =====================================================================
    % THRUSTER ACTUATOR MODEL (BANG-BANG CONTROL)
    % Simulates ON/OFF firing logic and propellant mass flow rate.
    % =====================================================================
    
    torque_real = zeros(3,1);
    
    % Deadband to prevent infinite firing for microscopic errors
    deadband = 0.005; % [Nm]
    
    % 1. BANG-BANG LOGIC
    for i = 1:3
        if torque_cmd(i) > deadband
            torque_real(i) = thruster_max_torque;
        elseif torque_cmd(i) < -deadband
            torque_real(i) = -thruster_max_torque;
        else
            torque_real(i) = 0.0;
        end
    end
    
    % 2. PROPELLANT CONSUMPTION BUDGET [kg/s]
    % Force = Torque / Arm. Mass flow = Force / (Isp * g0)
    total_force = sum(abs(torque_real)) / thruster_arm;
    mass_flow_rate = total_force / (thruster_Isp * g0);
    
end

== matlab function ADCS_GNC_Real_Simulation/Rigid Body Dynamics_1 ==
  data: torque input; q_dot output; omega input; q input; I_tensor input; I_inv input; omega_dot output
function [q_dot, omega_dot] = rigid_body_dynamics(torque, omega, q, I_tensor, I_inv)
% =========================================================================
% RIGID BODY ROTATIONAL DYNAMICS + QUATERNION KINEMATICS
% =========================================================================
% Purpose:
%   Simulate the rotational motion of the spacecraft.
%
% Inputs:
%   torque   : Applied body torque [Tx; Ty; Tz] [Nm]
%              expressed in BODY coordinates
%
%   omega    : Body angular velocity [p; q; r] [rad/s]
%              expressed in BODY coordinates
%
%   q        : Attitude quaternion [qw; qx; qy; qz]
%              BODY attitude with respect to ECI
%
%   I_tensor : Spacecraft inertia tensor [kg*m^2]
%
%   I_inv    : Inverse inertia tensor [1/(kg*m^2)]
%
% Outputs:
%   q_dot    : Quaternion derivative
%
%   omega_dot: Body angular acceleration [rad/s^2]
%
% =========================================================================
% Dynamic equation:
%
%   I * omega_dot + omega x (I*omega) = torque
%
% Therefore:
%
%   omega_dot = I^-1 * [torque - omega x (I*omega)]
%
% =========================================================================


% -------------------------------------------------------------------------
% 1. INITIALIZE OUTPUTS
% -------------------------------------------------------------------------

q_dot     = zeros(4,1);
omega_dot = zeros(3,1);


% -------------------------------------------------------------------------
% 2. NORMALIZE QUATERNION FOR KINEMATIC CALCULATION
% -------------------------------------------------------------------------
% Numerical integration can cause a small drift in quaternion norm.
%
% We normalize the quaternion before calculating q_dot.
% This does not change the physical attitude.

q_norm = norm(q);

if q_norm > 1e-12
    q_unit = q / q_norm;
else
    % Safety fallback
    q_unit = [1; 0; 0; 0];
end


% -------------------------------------------------------------------------
% 3. ANGULAR MOMENTUM
% -------------------------------------------------------------------------
% Angular momentum:
%
%   H = I * omega

H = I_tensor * omega;


% -------------------------------------------------------------------------
% 4. GYROSCOPIC CROSS PRODUCT
% -------------------------------------------------------------------------
% Calculate:
%
%   omega x H
%
% where:
%
%   H = I * omega

cross_omega_H = [ ...
    omega(2)*H(3) - omega(3)*H(2);
    omega(3)*H(1) - omega(1)*H(3);
    omega(1)*H(2) - omega(2)*H(1) ];


% -------------------------------------------------------------------------
% 5. EULER ROTATIONAL DYNAMICS
% -------------------------------------------------------------------------
% Equation:
%
%   I * omega_dot = torque - omega x (I*omega)
%
% Therefore:
%
%   omega_dot = I^-1 * [torque - omega x (I*omega)]

omega_dot = I_inv * ( ...
    torque - cross_omega_H );


% -------------------------------------------------------------------------
% 6. BODY ANGULAR RATES
% -------------------------------------------------------------------------
% The three components are:
%
%   omega = [p; q; r]

p = omega(1);
q_rate = omega(2);
r = omega(3);


% -------------------------------------------------------------------------
% 7. QUATERNION KINEMATICS
% -------------------------------------------------------------------------
% Quaternion convention:
%
%   q = [qw; qx; qy; qz]
%
% with body angular velocity:
%
%   omega = [p; q; r]
%
% Quaternion differential equation:
%
%   q_dot = 0.5 * Omega(omega) * q
%
% where:
%
%       [ 0  -p  -q  -r ]
%       [ p   0   r  -q ]
% Omega=[ q  -r   0   p ]
%       [ r   q  -p   0 ]

Omega_mat = [ ...
     0,     -p,      -q_rate, -r;
     p,      0,       r,      -q_rate;
     q_rate,-r,       0,       p;
     r,      q_rate, -p,       0 ];


% Quaternion derivative
q_dot = 0.5 * Omega_mat * q_unit;


% -------------------------------------------------------------------------
% 8. END
% -------------------------------------------------------------------------

end
